simulink model "example_Window_Uvalue"  (R2018b)
settings: Solver=ode45  StartTime=0  StopTime=6*3600  MaxStep=600  RelTol=1e-3  EnableMultiTasking=on
undefined symbols (not defined in the file): Dreifach, Wärmeschutzglas
libraries: carnot x4
settings Model: Creator=drhf  LastModifiedBy=drhf
settings DataIOCC: LimitDataPoints=on  SaveFormat=Array
settings OptimizationCC: DefaultParameterBehavior=Inlined  LifeSpan=inf
settings DebuggingCC: UnderspecifiedInitializationDetection=Classic  MergeDetectMultiDrivingBlocksExec=none  SolverPrmCheckMsg=warning  SFUnexpectedBacktrackingDiag=warning  SFNoUnconditionalDefaultTransitionDiag=warning  SFExecutionAtInitializationDiag=none
settings HardwareCC: ProdBitPerPointer=32  ProdBitPerSizeT=32  ProdBitPerPtrDiffT=32  ProdLargestAtomicFloat=None  ProdIntDivRoundTo=Undefined  ProdEndianess=Unspecified  ProdWordSize=32  ProdHWDeviceType=32-bit Generic
settings ModelReferenceCC: PropagateSignalLabelsOutOfModel=off
settings SFSimCC: SimUseLocalCustomCode=off
settings RTWCC: RTWUseLocalCustomCode=off
settings CodeAppCC: StateflowObjectComments=on
settings GRTTargetCC: TargetLangStandard=C89/C90 (ANSI)  GeneratePreprocessorConditionals=Disable all
settings ConfigComp: CovMetricSettings=dw  CovHtmlReporting=on  CovSaveCumulativeToWorkspaceVar=on  CovSaveSingleToWorkspaceVar=on  CovExternalEMLEnable=off

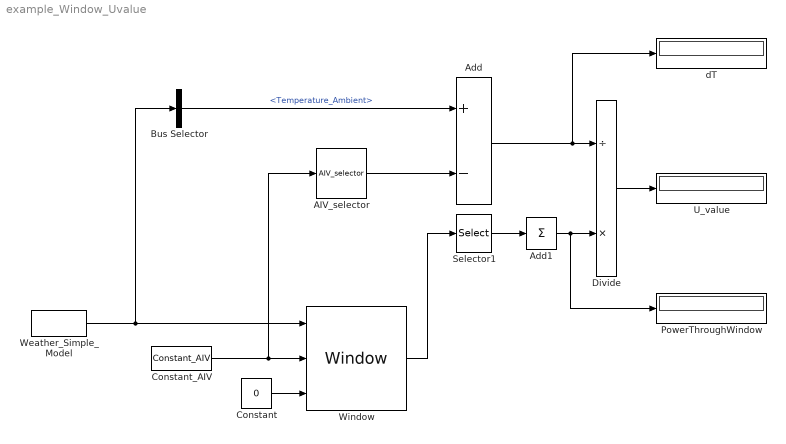
== system example_Window_Uvalue ==
  AIV_selector : carnot/Outputs/AIV_selector  e1=on  e2=off  e3=off  e4=off  e5=off  e6=off  e7=off  e8=off  e9=off
      settings: SourceProductName=Carnot
  Add : Sum  Inputs=+-
  Add1 : Sum  Inputs=1
  Bus Selector : BusSelector  OutputSignals=Temperature_Ambient
  Constant : Constant  Value=0
  Constant_AIV : carnot/Source/Ventilation/Constant_AIV  Tsens=20  Tcon=20  Trad=20  mw=0.012  mco=0.01  rhoair=1.2  cpair=1004  pair=100000  nair=0.5
      settings: SourceProductName=Carnot
  Divide : Product  Inputs=/*
  PowerThroughWindow : Display
  Selector1 : Selector  InputPortWidth=13  IndexOptions=Index vector (dialog)  Indices=[7 8]  OutputSizes=1
  U_value : Display
  Weather_Simple_Model : carnot/Weather/Weather_Simple_Model  Ibn=0  Idg=0  tamb=0  deltaTsky=0  rh=50  precip="10e-3/24/3600           % 10 mm in 24 h"  cloud=0.125  p=1013e2  vw=5.85  wdir=270  lat=60  colangle=0  colazi=0  colrot=0
      settings: SourceProductName=Carnot
  Window : carnot/Basic/Thermal_Models/Window  pos=180  windowsize=[1 1]  frame=0  Ug=1.8  gvalue=0.7  tauzero=0.8  numpanes=2  d=[0.004 0.004]  rho=[2500 2500]  cp="[1008  1008]"  t0=20  misc="[0.2,  0.1,  1,  1]"  shad_type=No shading  type_glazing=Dreifach-Wärmeschutzglas  tau_shad=0.01  bli_a=0.05  bli_b=1  bli_c=0.05  bli_d=0.05  bli_alpha=90  bli_refl=0.2
      settings: SourceProductName=Carnot
  dT : Display
  wires:
  Constant_AIV/1 -> AIV_selector/1, Window/2
  Window/1 -> Selector1/1
  AIV_selector/1 -> Add/2
  Add/1 -> dT/1, Divide/1
  Selector1/1 -> Add1/1
  Add1/1 -> PowerThroughWindow/1, Divide/2
  Divide/1 -> U_value/1
  Weather_Simple_Model/1 -> Window/1, Bus Selector/1
  Bus Selector/1 -> Add/1  "<Temperature_Ambient>"
  Constant/1 -> Window/3
